simulink model "mrefrobotarm_previous_y_previous_u_previous_ref_cex_3"  (R2018b)
settings: Solver=FixedStepAuto  StartTime=0.0  StopTime=20  RelTol=1e-3  AbsTol=1e-6
undefined symbols (not defined in the file or in its folder): cc, options
libraries: neural x396, simulink x2
(part 7 of 15)

== system mrefrobotarm_previous_y_previous_u_previous_ref_cex_3/cex_m2_adapt/Layer 3/Delays 1 ==
  "p{3}" : Inport  PortDimensions=30
      mask Display: e = 0.06;c1 = [120 230 180]/255;c2 = ([120 230 180]+0)/(256+128);c3 = ([120 230 180]+128)/(256+128);patch([0 1 1 0],[0 0 1 1],c1);patch([0 1 1 1-e 1-e 0+e],[0 0 1 1-e 0+e 0+e],c2);patch([0 0 1 1-e 0+e 0+e],[0 1 1 1-e 1-e 0+e],c3);plot([0 1 1 0 0],[0 0 1 1 0]);
  mux : Mux  Inputs=1
      mask Display: e = 0.06;c1 = [120 150 230]/255;c2 = ([120 150 230]+0)/383;c3 = ([120 150 230]+128)/383;patch([0 1 1 0],[0 0 1 1],c1);patch([0 1 1 1-e 1-e 0+e],[0 0 1 1-e 0+e 0+e],c2);patch([0 0 1 1-e 0+e 0+e],[0 1 1 1-e 1-e 0+e],c3);plot([0 1 1 0 0],[0 0 1 1 0]);disp('Mux')
  "pd{3,2}" : Outport
      mask Display: e = 0.06;c1 = [120 230 180]/255;c2 = ([120 230 180]+0)/(256+128);c3 = ([120 230 180]+128)/(256+128);patch([0 1 1 0],[0 0 1 1],c1);patch([0 1 1 1-e 1-e 0+e],[0 0 1 1-e 0+e 0+e],c2);patch([0 0 1 1-e 0+e 0+e],[0 1 1 1-e 1-e 0+e],c3);plot([0 1 1 0 0],[0 0 1 1 0]);
  wires:
  "p{3}"/1 -> mux/1
  mux/1 -> "pd{3,2}"/1

== system mrefrobotarm_previous_y_previous_u_previous_ref_cex_3/cex_m2_adapt/Layer 3/LW{3,2} ==
  "ad{3,2}" : Inport  PortDimensions=30
      mask Display: e = 0.06;c1 = [120 230 180]/255;c2 = ([120 230 180]+0)/(256+128);c3 = ([120 230 180]+128)/(256+128);patch([0 1 1 0],[0 0 1 1],c1);patch([0 1 1 1-e 1-e 0+e],[0 0 1 1-e 0+e 0+e],c2);patch([0 0 1 1-e 0+e 0+e],[0 1 1 1-e 1-e 0+e],c3);plot([0 1 1 0 0],[0 0 1 1 0]);
  "IW{3,2}(1,:)'" : Constant  Value=[-0.05505125570900899767412539631550316698849201202392578125;-0.32891261733908494502287567229359410703182220458984375;0.415382135802389473866469415952451527118682861328125;-0.2282730838579582754999108828997123055160045623779296875;0.166865414887934881971176537263090722262859344482421875;-0.28767207852958420755129509416292421519756317138671875;-0.321285823362595035490585360093973577022552490234375;0.1207160846177025848025010645869770087301731109619140625;-0.01460446132137031838293950158913503400981426239013671875;0.5016492750276049239488429520861245691776275634765625;0.357718762934432665812067853039479814469814300537109375;-0.006297882074193773827008868693155818618834018707275390625;-0.0450799800946801443313205481899785809218883514404296875;0.0099702407715112732755624591618470731191337108612060546875;0.285267027442495102462771683349274098873138427734375;0.2491387260000068604171019615023396909236907958984375;-0.1838273412419492991443092932968284003436565399169921875;0.459873080865493555347001120026106946170330047607421875;0.036965404262347324737536524708048091270029544830322265625;0.038819216468767563099628858935830066911876201629638671875;0.320204321153936266597384019405581057071685791015625;-0.0222015075110175881534235742265082080848515033721923828125;0.1764216096534496347469911370353656820952892303466796875;-0.36905645815071663751183450585813261568546295166015625;-0.029660070230276454339435332485663820989429950714111328125;-0.036545858611714283903371125461490009911358356475830078125;0.2780670093635304596091373241506516933441162109375;0.5598975676846238425099500091164372861385345458984375;-0.217836892233410794883496919283061288297176361083984375;0.406407184848614377870035241357982158660888671875]
      mask Display: e = 0.06;c1 = [120 150 230]/255;c2 = ([120 150 230]+0)/383;c3 = ([120 150 230]+128)/383;patch([0 1 1 0],[0 0 1 1],c1);patch([0 1 1 1-e 1-e 0+e],[0 0 1 1-e 0+e 0+e],c2);patch([0 0 1 1-e 0+e 0+e],[0 1 1 1-e 1-e 0+e],c3);plot([0 1 1 0 0],[0 0 1 1 0]);disp('weights');
  Mux : Mux  Inputs=1
      mask Display: e = 0.06;c1 = [120 150 230]/255;c2 = ([120 150 230]+0)/383;c3 = ([120 150 230]+128)/383;patch([0 1 1 0],[0 0 1 1],c1);patch([0 1 1 1-e 1-e 0+e],[0 0 1 1-e 0+e 0+e],c2);patch([0 0 1 1-e 0+e 0+e],[0 1 1 1-e 1-e 0+e],c3);plot([0 1 1 0 0],[0 0 1 1 0]);disp('Mux');
  dotprod1 : neural/Weight Functions/dotprod
  "lz{3,2}" : Outport
      mask Display: e = 0.06;c1 = [120 230 180]/255;c2 = ([120 230 180]+0)/(256+128);c3 = ([120 230 180]+128)/(256+128);patch([0 1 1 0],[0 0 1 1],c1);patch([0 1 1 1-e 1-e 0+e],[0 0 1 1-e 0+e 0+e],c2);patch([0 0 1 1-e 0+e 0+e],[0 1 1 1-e 1-e 0+e],c3);plot([0 1 1 0 0],[0 0 1 1 0]);
  wires:
  "IW{3,2}(1,:)'"/1 -> dotprod1/1
  "ad{3,2}"/1 -> dotprod1/2
  dotprod1/1 -> Mux/1
  Mux/1 -> "lz{3,2}"/1

== system mrefrobotarm_previous_y_previous_u_previous_ref_cex_3/cex_m3_adapt/Layer 1/Delays 1 ==
  "p{1}" : Inport  PortDimensions=10
      mask Display: e = 0.06;c1 = [120 230 180]/255;c2 = ([120 230 180]+0)/(256+128);c3 = ([120 230 180]+128)/(256+128);patch([0 1 1 0],[0 0 1 1],c1);patch([0 1 1 1-e 1-e 0+e],[0 0 1 1-e 0+e 0+e],c2);patch([0 0 1 1-e 0+e 0+e],[0 1 1 1-e 1-e 0+e],c3);plot([0 1 1 0 0],[0 0 1 1 0]);
  mux : Mux  Inputs=1
      mask Display: e = 0.06;c1 = [120 150 230]/255;c2 = ([120 150 230]+0)/383;c3 = ([120 150 230]+128)/383;patch([0 1 1 0],[0 0 1 1],c1);patch([0 1 1 1-e 1-e 0+e],[0 0 1 1-e 0+e 0+e],c2);patch([0 0 1 1-e 0+e 0+e],[0 1 1 1-e 1-e 0+e],c3);plot([0 1 1 0 0],[0 0 1 1 0]);disp('Mux')
  "pd{1,1}" : Outport
      mask Display: e = 0.06;c1 = [120 230 180]/255;c2 = ([120 230 180]+0)/(256+128);c3 = ([120 230 180]+128)/(256+128);patch([0 1 1 0],[0 0 1 1],c1);patch([0 1 1 1-e 1-e 0+e],[0 0 1 1-e 0+e 0+e],c2);patch([0 0 1 1-e 0+e 0+e],[0 1 1 1-e 1-e 0+e],c3);plot([0 1 1 0 0],[0 0 1 1 0]);
  wires:
  "p{1}"/1 -> mux/1
  mux/1 -> "pd{1,1}"/1

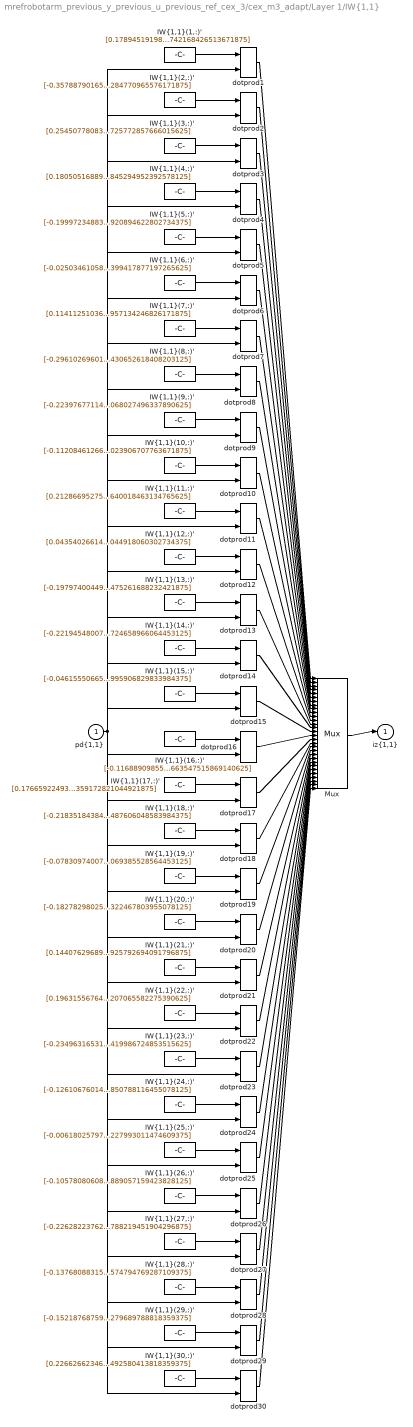
== system mrefrobotarm_previous_y_previous_u_previous_ref_cex_3/cex_m3_adapt/Layer 1/IW{1,1} ==
  "pd{1,1}" : Inport  PortDimensions=10
      mask Display: e = 0.06;c1 = [120 230 180]/255;c2 = ([120 230 180]+0)/(256+128);c3 = ([120 230 180]+128)/(256+128);patch([0 1 1 0],[0 0 1 1],c1);patch([0 1 1 1-e 1-e 0+e],[0 0 1 1-e 0+e 0+e],c2);patch([0 0 1 1-e 0+e 0+e],[0 1 1 1-e 1-e 0+e],c3);plot([0 1 1 0 0],[0 0 1 1 0]);
  "IW{1,1}(1,:)'" : Constant  Value=[0.178945191981768558786569656149367801845073699951171875;0.0268084580163748913139709628694618004374206066131591796875;-0.01942320989874750380987933340293238870799541473388671875;-0.08160193884960249832705159178658504970371723175048828125;-0.09141040548628250050899879397547920234501361846923828125;-0.03003006458415546919837879613623954355716705322265625;-0.2824185437874746629205446879495866596698760986328125;0.13111273715930271688279162844992242753505706787109375;-0.18958976093589396949568026684573851525783538818359375;0.2425037970369951778604189485122333280742168426513671875]
      mask Display: e = 0.06;c1 = [120 150 230]/255;c2 = ([120 150 230]+0)/383;c3 = ([120 150 230]+128)/383;patch([0 1 1 0],[0 0 1 1],c1);patch([0 1 1 1-e 1-e 0+e],[0 0 1 1-e 0+e 0+e],c2);patch([0 0 1 1-e 0+e 0+e],[0 1 1 1-e 1-e 0+e],c3);plot([0 1 1 0 0],[0 0 1 1 0]);disp('Weights');
  "IW{1,1}(10,:)'" : Constant  Value=[-0.11208461266883167073427074456049012951552867889404296875;0.357118226286030460148168685918790288269519805908203125;-0.2471912861743887079857273647576221264898777008056640625;0.02694087701823717762028564948195707984268665313720703125;0.333344688343605366487309993317467160522937774658203125;-0.3923720531710868097974298507324419915676116943359375;0.10448361375716642973632275470663444139063358306884765625;-0.06700094235100791106862772039676201529800891876220703125;-0.0864068226303956465894628991009085439145565032958984375;-0.39109116979221425491886066083679907023906707763671875]
      mask Display: e = 0.06;c1 = [120 150 230]/255;c2 = ([120 150 230]+0)/383;c3 = ([120 150 230]+128)/383;patch([0 1 1 0],[0 0 1 1],c1);patch([0 1 1 1-e 1-e 0+e],[0 0 1 1-e 0+e 0+e],c2);patch([0 0 1 1-e 0+e 0+e],[0 1 1 1-e 1-e 0+e],c3);plot([0 1 1 0 0],[0 0 1 1 0]);disp('Weights');
  "IW{1,1}(11,:)'" : Constant  Value=[0.2128669527513860348921781451281276531517505645751953125;-0.2022164608257241702471418420827831141650676727294921875;0.024891361043484862280994462935268529690802097320556640625;-0.1523659720349933854866009141915128566324710845947265625;0.01343407208234892631637524829102403600700199604034423828125;0.333788117058362920896996683950419537723064422607421875;-0.12203835126155791745983236751271761022508144378662109375;0.154459927321787870990732471909723244607448577880859375;-0.0299672295637235762411076933631193242035806179046630859375;0.1513977074327107763540567475502029992640018463134765625]
      mask Display: e = 0.06;c1 = [120 150 230]/255;c2 = ([120 150 230]+0)/383;c3 = ([120 150 230]+128)/383;patch([0 1 1 0],[0 0 1 1],c1);patch([0 1 1 1-e 1-e 0+e],[0 0 1 1-e 0+e 0+e],c2);patch([0 0 1 1-e 0+e 0+e],[0 1 1 1-e 1-e 0+e],c3);plot([0 1 1 0 0],[0 0 1 1 0]);disp('Weights');
  "IW{1,1}(12,:)'" : Constant  Value=[0.043540266140519097437522333393644657917320728302001953125;-0.41452389872784956015294710596208460628986358642578125;0.2152802602883765181740471916782553307712078094482421875;0.1665741110113748979504322278444305993616580963134765625;-0.02357125033996217144949270050346967764198780059814453125;0.0857396390633823612947850278942496515810489654541015625;-0.195803542101584737711306161145330406725406646728515625;-0.1624956920043294505973108243779279291629791259765625;0.251216496349794427001000940435915254056453704833984375;-0.10692808582410960605013627855441882275044918060302734375]
      mask Display: e = 0.06;c1 = [120 150 230]/255;c2 = ([120 150 230]+0)/383;c3 = ([120 150 230]+128)/383;patch([0 1 1 0],[0 0 1 1],c1);patch([0 1 1 1-e 1-e 0+e],[0 0 1 1-e 0+e 0+e],c2);patch([0 0 1 1-e 0+e 0+e],[0 1 1 1-e 1-e 0+e],c3);plot([0 1 1 0 0],[0 0 1 1 0]);disp('Weights');
  "IW{1,1}(13,:)'" : Constant  Value=[-0.197974004496612343562134128660545684397220611572265625;0.1845410275017112244899664119657245464622974395751953125;-0.06383715487094511475962832491859444417059421539306640625;0.212121113393368199151467479168786667287349700927734375;-0.13808972121742824068491017897031269967555999755859375;0.038970279682366611162525060763073270209133625030517578125;0.105618059669576991321804371182224713265895843505859375;-0.1502222390986265032619684234305168502032756805419921875;-0.24632715103327262884391757324920035898685455322265625;0.2171770229910456873057000848348252475261688232421875]
      mask Display: e = 0.06;c1 = [120 150 230]/255;c2 = ([120 150 230]+0)/383;c3 = ([120 150 230]+128)/383;patch([0 1 1 0],[0 0 1 1],c1);patch([0 1 1 1-e 1-e 0+e],[0 0 1 1-e 0+e 0+e],c2);patch([0 0 1 1-e 0+e 0+e],[0 1 1 1-e 1-e 0+e],c3);plot([0 1 1 0 0],[0 0 1 1 0]);disp('Weights');
  "IW{1,1}(14,:)'" : Constant  Value=[-0.2219454800708457742342005758473533205687999725341796875;-0.0314615502081657949506876548184663988649845123291015625;0.251007339093214987268964932809467427432537078857421875;-0.0716759461367137695742002279075677506625652313232421875;-0.0172769229951700541147996403879005811177194118499755859375;0.1873159588626435445579687666395329870283603668212890625;0.190073886084198784285348438061191700398921966552734375;0.256287607810354589599199925942230038344860076904296875;-0.12311553026235876051597273317383951507508754730224609375;0.08368773604129982335297910367444274015724658966064453125]
      mask Display: e = 0.06;c1 = [120 150 230]/255;c2 = ([120 150 230]+0)/383;c3 = ([120 150 230]+128)/383;patch([0 1 1 0],[0 0 1 1],c1);patch([0 1 1 1-e 1-e 0+e],[0 0 1 1-e 0+e 0+e],c2);patch([0 0 1 1-e 0+e 0+e],[0 1 1 1-e 1-e 0+e],c3);plot([0 1 1 0 0],[0 0 1 1 0]);disp('Weights');
  "IW{1,1}(15,:)'" : Constant  Value=[-0.046155506650369430843294793476161430589854717254638671875;-0.1501346179631337929283318999296170659363269805908203125;0.0092307094765049883811069975081409211270511150360107421875;-0.263036000331381802919139545338111929595470428466796875;-0.2327975024204980425412969680110109038650989532470703125;-0.2026112126291482462558946053832187317311763763427734375;0.051737301403803448440754664261476136744022369384765625;-0.209756826452610234401419120331411249935626983642578125;0.1810701775696283988281720667146146297454833984375;-0.037977678064883800546081005222731619141995906829833984375]
      mask Display: e = 0.06;c1 = [120 150 230]/255;c2 = ([120 150 230]+0)/383;c3 = ([120 150 230]+128)/383;patch([0 1 1 0],[0 0 1 1],c1);patch([0 1 1 1-e 1-e 0+e],[0 0 1 1-e 0+e 0+e],c2);patch([0 0 1 1-e 0+e 0+e],[0 1 1 1-e 1-e 0+e],c3);plot([0 1 1 0 0],[0 0 1 1 0]);disp('Weights');
  "IW{1,1}(16,:)'" : Constant  Value=[-0.11688909855486113997802277708615292795002460479736328125;0.1948288754210096562768939065790618769824504852294921875;0.245145418046943730505660141716361977159976959228515625;0.06314581600642978076454170377473928965628147125244140625;-0.1710702295590592336704816034398390911519527435302734375;0.2286371699946944946457705327702569775283336639404296875;0.1679562205641119965182639361955807544291019439697265625;-0.136021170064964225243642204077332280576229095458984375;0.1710849460743354699676643804195919074118137359619140625;-0.035177187616954430637861150898970663547515869140625]
      mask Display: e = 0.06;c1 = [120 150 230]/255;c2 = ([120 150 230]+0)/383;c3 = ([120 150 230]+128)/383;patch([0 1 1 0],[0 0 1 1],c1);patch([0 1 1 1-e 1-e 0+e],[0 0 1 1-e 0+e 0+e],c2);patch([0 0 1 1-e 0+e 0+e],[0 1 1 1-e 1-e 0+e],c3);plot([0 1 1 0 0],[0 0 1 1 0]);disp('Weights');
  "IW{1,1}(17,:)'" : Constant  Value=[0.1766592249333858999360558073021820746362209320068359375;-0.079243523014492278644382849961402826011180877685546875;-0.0793114419622731048331587544453213922679424285888671875;-0.1959259597757977700016596145360381342470645904541015625;0.11564958667334186703801179874062654562294483184814453125;0.0078762918190796345208060103004754637368023395538330078125;0.042690054177657914269428118814175832085311412811279296875;-0.209400363475176154448575971400714479386806488037109375;-0.1737241496218795144823587861537816934287548065185546875;-0.30776352047767552289059267422999255359172821044921875]
      mask Display: e = 0.06;c1 = [120 150 230]/255;c2 = ([120 150 230]+0)/383;c3 = ([120 150 230]+128)/383;patch([0 1 1 0],[0 0 1 1],c1);patch([0 1 1 1-e 1-e 0+e],[0 0 1 1-e 0+e 0+e],c2);patch([0 0 1 1-e 0+e 0+e],[0 1 1 1-e 1-e 0+e],c3);plot([0 1 1 0 0],[0 0 1 1 0]);disp('Weights');
  "IW{1,1}(18,:)'" : Constant  Value=[-0.21835184384607442265036070239148102700710296630859375;0.06422592695237487603332482422047178260982036590576171875;-0.061954335238517045658657167450655833818018436431884765625;0.09804573861090604136592219219892285764217376708984375;-0.1940740141485696457213094845428713597357273101806640625;0.1005519891302661117382655220353626646101474761962890625;0.05512324942271966399243154910436714999377727508544921875;-0.2225722743997785302294545317636220715939998626708984375;0.3076953257419956511142800081870518624782562255859375;0.03510283654959012178409238913445733487606048583984375]
      mask Display: e = 0.06;c1 = [120 150 230]/255;c2 = ([120 150 230]+0)/383;c3 = ([120 150 230]+128)/383;patch([0 1 1 0],[0 0 1 1],c1);patch([0 1 1 1-e 1-e 0+e],[0 0 1 1-e 0+e 0+e],c2);patch([0 0 1 1-e 0+e 0+e],[0 1 1 1-e 1-e 0+e],c3);plot([0 1 1 0 0],[0 0 1 1 0]);disp('Weights');
  "IW{1,1}(19,:)'" : Constant  Value=[-0.07830974007872003317398679200778133235871791839599609375;-0.11016442094929913830814172115424298681318759918212890625;0.0703650635811621516513270080395159311592578887939453125;-0.07372103454447127834914255117837456054985523223876953125;0.24983208769968501261615756448009051382541656494140625;-0.144793585299214433437242632862762548029422760009765625;0.321295391447031286613622569348081015050411224365234375;0.01420628885393082109500628718024017871357500553131103515625;-0.20975856453201091600391237079747952520847320556640625;-0.13789742091780443633552977189538069069385528564453125]
      mask Display: e = 0.06;c1 = [120 150 230]/255;c2 = ([120 150 230]+0)/383;c3 = ([120 150 230]+128)/383;patch([0 1 1 0],[0 0 1 1],c1);patch([0 1 1 1-e 1-e 0+e],[0 0 1 1-e 0+e 0+e],c2);patch([0 0 1 1-e 0+e 0+e],[0 1 1 1-e 1-e 0+e],c3);plot([0 1 1 0 0],[0 0 1 1 0]);disp('Weights');
  "IW{1,1}(2,:)'" : Constant  Value=[-0.357887901653798190526600819794111885130405426025390625;-0.1701515671788660366559042813605628907680511474609375;0.1283989037480392225720748911044211126863956451416015625;0.02788164361507915189886119833317934535443782806396484375;0.2413361422270965395142638953984715044498443603515625;-0.088300044465701998941398187525919638574123382568359375;-0.059645869356086879398137767793741659261286258697509765625;-0.1817714760329936229954483906112727709114551544189453125;-0.2027513482131242106287771775896544568240642547607421875;0.0361216702772399755883014904611627571284770965576171875]
      mask Display: e = 0.06;c1 = [120 150 230]/255;c2 = ([120 150 230]+0)/383;c3 = ([120 150 230]+128)/383;patch([0 1 1 0],[0 0 1 1],c1);patch([0 1 1 1-e 1-e 0+e],[0 0 1 1-e 0+e 0+e],c2);patch([0 0 1 1-e 0+e 0+e],[0 1 1 1-e 1-e 0+e],c3);plot([0 1 1 0 0],[0 0 1 1 0]);disp('Weights');
  "IW{1,1}(20,:)'" : Constant  Value=[-0.1827829802579581663923846690522623248398303985595703125;0.429762651162807263194309825848904438316822052001953125;0.047505038489587501915334399882340221665799617767333984375;-0.051722345762055088602693331267801113426685333251953125;0.09193146508099292457671936062979511916637420654296875;-0.378843620454603124958481430439860559999942779541015625;-0.0326607967189324333023847657386795617640018463134765625;-0.035941474259534145208050404107780195772647857666015625;-0.0821945981870604303054506090120412409305572509765625;-0.1229102528711117081616777113595162518322467803955078125]
      mask Display: e = 0.06;c1 = [120 150 230]/255;c2 = ([120 150 230]+0)/383;c3 = ([120 150 230]+128)/383;patch([0 1 1 0],[0 0 1 1],c1);patch([0 1 1 1-e 1-e 0+e],[0 0 1 1-e 0+e 0+e],c2);patch([0 0 1 1-e 0+e 0+e],[0 1 1 1-e 1-e 0+e],c3);plot([0 1 1 0 0],[0 0 1 1 0]);disp('Weights');
  "IW{1,1}(21,:)'" : Constant  Value=[0.1440762968925218545646060874787508510053157806396484375;0.0567506407928204670287897215530392713844776153564453125;0.18700116751710360585292391988332383334636688232421875;-0.1647839415001810803307336072975886054337024688720703125;-0.237372168308809750048027353841462172567844390869140625;0.253696421920278913919588603675947524607181549072265625;-0.2346470875872900541114773886874900199472904205322265625;0.0215979693524790301861759900248216581530869007110595703125;0.23838840468809874284517036358010955154895782470703125;-0.0025999808583438833824164060359862560289911925792694091796875]
      mask Display: e = 0.06;c1 = [120 150 230]/255;c2 = ([120 150 230]+0)/383;c3 = ([120 150 230]+128)/383;patch([0 1 1 0],[0 0 1 1],c1);patch([0 1 1 1-e 1-e 0+e],[0 0 1 1-e 0+e 0+e],c2);patch([0 0 1 1-e 0+e 0+e],[0 1 1 1-e 1-e 0+e],c3);plot([0 1 1 0 0],[0 0 1 1 0]);disp('Weights');
  "IW{1,1}(22,:)'" : Constant  Value=[0.1963155676454732267988134708502911962568759918212890625;-0.052000800150651706188487111148788244463503360748291015625;-0.271534817188853139224846700017224065959453582763671875;-0.0895242263296035234443337458287714980542659759521484375;-0.03695111731571724955625057873476180247962474822998046875;0.004478426352357927318903474400713093928061425685882568359375;0.259203736873355072845015456550754606723785400390625;-0.08894384724343833148463289717255975119769573211669921875;0.0322689444357559251930211985381902195513248443603515625;0.306951155849270629349945238573127426207065582275390625]
      mask Display: e = 0.06;c1 = [120 150 230]/255;c2 = ([120 150 230]+0)/383;c3 = ([120 150 230]+128)/383;patch([0 1 1 0],[0 0 1 1],c1);patch([0 1 1 1-e 1-e 0+e],[0 0 1 1-e 0+e 0+e],c2);patch([0 0 1 1-e 0+e 0+e],[0 1 1 1-e 1-e 0+e],c3);plot([0 1 1 0 0],[0 0 1 1 0]);disp('Weights');
  "IW{1,1}(23,:)'" : Constant  Value=[-0.2349631653173517020771754459929070435464382171630859375;-0.17641432489103936465113520171144045889377593994140625;0.234912163501337811766234153765253722667694091796875;0.09797598509365797181391855019683134742081165313720703125;0.27541255175971579571836400646134279668331146240234375;-0.006673026099757165506554112965886815800331532955169677734375;-0.08630883651204894480013507518378901295363903045654296875;-0.0492544357827646994696380033929017372429370880126953125;0.3119811671615313475314223978784866631031036376953125;-0.1301709266317944424518060486661852337419986724853515625]
      mask Display: e = 0.06;c1 = [120 150 230]/255;c2 = ([120 150 230]+0)/383;c3 = ([120 150 230]+128)/383;patch([0 1 1 0],[0 0 1 1],c1);patch([0 1 1 1-e 1-e 0+e],[0 0 1 1-e 0+e 0+e],c2);patch([0 0 1 1-e 0+e 0+e],[0 1 1 1-e 1-e 0+e],c3);plot([0 1 1 0 0],[0 0 1 1 0]);disp('Weights');
  "IW{1,1}(24,:)'" : Constant  Value=[-0.126106760142745744079917358249076642096042633056640625;0.08453625577713620720121667773128137923777103424072265625;-0.1709608100596076152299929162836633622646331787109375;0.291185745152728825413390723042539320886135101318359375;0.11522508174914349032835758634973899461328983306884765625;0.270251365920760211469797695826855488121509552001953125;0.11501887877284679151390633933260687626898288726806640625;0.068932792124765829289145813163486309349536895751953125;0.0923120543919047076286688024993054568767547607421875;0.12574612443187327404103825756465084850788116455078125]
      mask Display: e = 0.06;c1 = [120 150 230]/255;c2 = ([120 150 230]+0)/383;c3 = ([120 150 230]+128)/383;patch([0 1 1 0],[0 0 1 1],c1);patch([0 1 1 1-e 1-e 0+e],[0 0 1 1-e 0+e 0+e],c2);patch([0 0 1 1-e 0+e 0+e],[0 1 1 1-e 1-e 0+e],c3);plot([0 1 1 0 0],[0 0 1 1 0]);disp('Weights');
  "IW{1,1}(25,:)'" : Constant  Value=[-0.00618025797029859470799184606448761769570410251617431640625;0.1585465053945979418958955875496030785143375396728515625;0.1885969000154264219037969496639561839401721954345703125;-0.0168828019608085848346501478545178542844951152801513671875;-0.1887944529566672191567278105139848776161670684814453125;0.127242314587684257620736616445356048643589019775390625;-0.0185715628598672015392434531122489715926349163055419921875;0.271969474158978596900482216369709931313991546630859375;0.11406243308473180964046633789621409960091114044189453125;-0.2380937855451320250832480951430625282227993011474609375]
      mask Display: e = 0.06;c1 = [120 150 230]/255;c2 = ([120 150 230]+0)/383;c3 = ([120 150 230]+128)/383;patch([0 1 1 0],[0 0 1 1],c1);patch([0 1 1 1-e 1-e 0+e],[0 0 1 1-e 0+e 0+e],c2);patch([0 0 1 1-e 0+e 0+e],[0 1 1 1-e 1-e 0+e],c3);plot([0 1 1 0 0],[0 0 1 1 0]);disp('Weights');
  "IW{1,1}(26,:)'" : Constant  Value=[-0.1057808060816034234630222954365308396518230438232421875;0.1781977064655418108163331680771079845726490020751953125;-0.25777667563861805799518833737238310277462005615234375;-0.12119534915408673725334409709830651991069316864013671875;0.107985561966510490439219438485451973974704742431640625;0.032407409608050032068238266447224305011332035064697265625;0.233920314605909063221389487807755358517169952392578125;0.04861961739534488569081105424629640765488147735595703125;-0.07777090296223808374431740730869933031499385833740234375;-0.06606828886995681771043820162958581931889057159423828125]
      mask Display: e = 0.06;c1 = [120 150 230]/255;c2 = ([120 150 230]+0)/383;c3 = ([120 150 230]+128)/383;patch([0 1 1 0],[0 0 1 1],c1);patch([0 1 1 1-e 1-e 0+e],[0 0 1 1-e 0+e 0+e],c2);patch([0 0 1 1-e 0+e 0+e],[0 1 1 1-e 1-e 0+e],c3);plot([0 1 1 0 0],[0 0 1 1 0]);disp('Weights');
  "IW{1,1}(27,:)'" : Constant  Value=[-0.2262822376263129708906518544608843512833118438720703125;0.228376340453633808191824527966673485934734344482421875;-0.04633621010046702626272718816835549660027027130126953125;-0.21557195704307108297115291861700825393199920654296875;-0.024477301255473281338392865791320218704640865325927734375;-0.061316063341058886504431058028785628266632556915283203125;0.19263265023581077617365053811226971447467803955078125;0.21379549598064950810538675796124152839183807373046875;0.2402192329457557284921875861982698552310466766357421875;0.004684371003340066612341541230080110835842788219451904296875]
      mask Display: e = 0.06;c1 = [120 150 230]/255;c2 = ([120 150 230]+0)/383;c3 = ([120 150 230]+128)/383;patch([0 1 1 0],[0 0 1 1],c1);patch([0 1 1 1-e 1-e 0+e],[0 0 1 1-e 0+e 0+e],c2);patch([0 0 1 1-e 0+e 0+e],[0 1 1 1-e 1-e 0+e],c3);plot([0 1 1 0 0],[0 0 1 1 0]);disp('Weights');
  "IW{1,1}(28,:)'" : Constant  Value=[-0.137680883158168343438632064135163091123104095458984375;0.1357222867627534690360135982700739987194538116455078125;0.10901823944261945786848855277639813721179962158203125;-0.0209386438839303558323567955312682897783815860748291015625;0.1596112896660535629411725722093251533806324005126953125;-0.224640567202143426328575515071861445903778076171875;-0.126750799819497272924451181097538210451602935791015625;0.1520166458419669186508116354161757044494152069091796875;0.21814044502030494054878317911061458289623260498046875;-0.04722597981823682677937625840058899484574794769287109375]
      mask Display: e = 0.06;c1 = [120 150 230]/255;c2 = ([120 150 230]+0)/383;c3 = ([120 150 230]+128)/383;patch([0 1 1 0],[0 0 1 1],c1);patch([0 1 1 1-e 1-e 0+e],[0 0 1 1-e 0+e 0+e],c2);patch([0 0 1 1-e 0+e 0+e],[0 1 1 1-e 1-e 0+e],c3);plot([0 1 1 0 0],[0 0 1 1 0]);disp('Weights');
  "IW{1,1}(29,:)'" : Constant  Value=[-0.152187687592834297589661218808032572269439697265625;-0.045824332750618645970774878151132725179195404052734375;0.0755527612060038489261160066234879195690155029296875;-0.185261645573886746252156854097847826778888702392578125;0.1512516263026323082296897837295546196401119232177734375;-0.1412085300290002454204341120203025639057159423828125;-0.0868175921655288396205918388659483753144741058349609375;-0.2248728415417697579226086190828937105834484100341796875;-0.1651996539641483463523030650321743451058864593505859375;0.15755372160029990080687412046245299279689788818359375]
      mask Display: e = 0.06;c1 = [120 150 230]/255;c2 = ([120 150 230]+0)/383;c3 = ([120 150 230]+128)/383;patch([0 1 1 0],[0 0 1 1],c1);patch([0 1 1 1-e 1-e 0+e],[0 0 1 1-e 0+e 0+e],c2);patch([0 0 1 1-e 0+e 0+e],[0 1 1 1-e 1-e 0+e],c3);plot([0 1 1 0 0],[0 0 1 1 0]);disp('Weights');
  "IW{1,1}(3,:)'" : Constant  Value=[0.2545077808367981475612396025098860263824462890625;0.040200788949858144716298369303331128321588039398193359375;0.16885529405137200686937148930155672132968902587890625;0.2275439655005222217010185659091803245246410369873046875;0.238416395262542712973896641415194608271121978759765625;0.1413290820820835846927110424076090566813945770263671875;0.10575858892024310453638946682985988445580005645751953125;0.13340769511394778845669861766509711742401123046875;0.12030518096117114035248363279606564901769161224365234375;0.1159861633997042729138371441877097822725772857666015625]
      mask Display: e = 0.06;c1 = [120 150 230]/255;c2 = ([120 150 230]+0)/383;c3 = ([120 150 230]+128)/383;patch([0 1 1 0],[0 0 1 1],c1);patch([0 1 1 1-e 1-e 0+e],[0 0 1 1-e 0+e 0+e],c2);patch([0 0 1 1-e 0+e 0+e],[0 1 1 1-e 1-e 0+e],c3);plot([0 1 1 0 0],[0 0 1 1 0]);disp('Weights');
  "IW{1,1}(30,:)'" : Constant  Value=[0.2266266234642653198960715599241666495800018310546875;0.1400900685113556087824093765448196791112422943115234375;-0.111869786415829397530075084432610310614109039306640625;0.2012524327790981004682180355302989482879638671875;-0.0186272552060192768397239859723413246683776378631591796875;-0.2006401151986405839711125054236617870628833770751953125;-0.09615820230093363729650945970206521451473236083984375;-0.1772150327736468355954713160826941020786762237548828125;0.031918350708111407898481814982005744241178035736083984375;0.26696557032662437958236978374770842492580413818359375]
      mask Display: e = 0.06;c1 = [120 150 230]/255;c2 = ([120 150 230]+0)/383;c3 = ([120 150 230]+128)/383;patch([0 1 1 0],[0 0 1 1],c1);patch([0 1 1 1-e 1-e 0+e],[0 0 1 1-e 0+e 0+e],c2);patch([0 0 1 1-e 0+e 0+e],[0 1 1 1-e 1-e 0+e],c3);plot([0 1 1 0 0],[0 0 1 1 0]);disp('Weights');
  "IW{1,1}(4,:)'" : Constant  Value=[0.1805051688978105695060349944469635374844074249267578125;-0.2288494814434568758176880010068998672068119049072265625;0.1818720593742958191452174787627882324159145355224609375;-0.037942953544057432535563378905862919054925441741943359375;-0.005389968593745760212787576648452159133739769458770751953125;0.1827951113605962019104111959677538834512233734130859375;-0.055292178726246830888779726365100941620767116546630859375;-0.14743556348991282423099846710101701319217681884765625;-0.2793310799565957847079289422254078090190887451171875;0.1322500450627073498299779430453781969845294952392578125]
      mask Display: e = 0.06;c1 = [120 150 230]/255;c2 = ([120 150 230]+0)/383;c3 = ([120 150 230]+128)/383;patch([0 1 1 0],[0 0 1 1],c1);patch([0 1 1 1-e 1-e 0+e],[0 0 1 1-e 0+e 0+e],c2);patch([0 0 1 1-e 0+e 0+e],[0 1 1 1-e 1-e 0+e],c3);plot([0 1 1 0 0],[0 0 1 1 0]);disp('Weights');
  "IW{1,1}(5,:)'" : Constant  Value=[-0.1999723488349300082322912430754513479769229888916015625;-0.16296175086491249128783920241403393447399139404296875;-0.10880631133516142916572988497136975638568401336669921875;0.051130749748494554174360615661498741246759891510009765625;-0.02372298130379191238858993528992868959903717041015625;0.0517192502525367914234522004335303790867328643798828125;-0.1720233138208674128488695487249060533940792083740234375;-0.204481799674667341637501749573857523500919342041015625;0.1663037664222504485866949153205496259033679962158203125;-0.139186530375922268287780525497510097920894622802734375]
      mask Display: e = 0.06;c1 = [120 150 230]/255;c2 = ([120 150 230]+0)/383;c3 = ([120 150 230]+128)/383;patch([0 1 1 0],[0 0 1 1],c1);patch([0 1 1 1-e 1-e 0+e],[0 0 1 1-e 0+e 0+e],c2);patch([0 0 1 1-e 0+e 0+e],[0 1 1 1-e 1-e 0+e],c3);plot([0 1 1 0 0],[0 0 1 1 0]);disp('Weights');
  "IW{1,1}(6,:)'" : Constant  Value=[-0.0250346105868364705859807628485214081592857837677001953125;-0.004457760763241335431883438644717898569069802761077880859375;0.0664046720124821521213931418969877995550632476806640625;-0.2130593218179563930192443876876495778560638427734375;0.1292973325083253133271909973700530827045440673828125;-0.1347766108497021608769728118204511702060699462890625;-0.235986082534269503430124359510955400764942169189453125;-0.0652885071425104157594176967904786579310894012451171875;-0.1443016385971503112717329031511326320469379425048828125;0.08876763803892606663481501527712680399417877197265625]
      mask Display: e = 0.06;c1 = [120 150 230]/255;c2 = ([120 150 230]+0)/383;c3 = ([120 150 230]+128)/383;patch([0 1 1 0],[0 0 1 1],c1);patch([0 1 1 1-e 1-e 0+e],[0 0 1 1-e 0+e 0+e],c2);patch([0 0 1 1-e 0+e 0+e],[0 1 1 1-e 1-e 0+e],c3);plot([0 1 1 0 0],[0 0 1 1 0]);disp('Weights');
  "IW{1,1}(7,:)'" : Constant  Value=[0.1141125103679923313837463183517684228718280792236328125;-0.071976397782599510488665828233934007585048675537109375;0.2194208546389509739693579604136175476014614105224609375;0.2087203652399640396719604495956446044147014617919921875;0.04279122020650989732803992637855117209255695343017578125;0.0121936683836014019000071328946432913653552532196044921875;0.10314941535816808670933397706903633661568164825439453125;0.215596517802053522228078463740530423820018768310546875;-0.11201446245962991266065245099525782279670238494873046875;0.267689612477664595768800381847540847957134246826171875]
      mask Display: e = 0.06;c1 = [120 150 230]/255;c2 = ([120 150 230]+0)/383;c3 = ([120 150 230]+128)/383;patch([0 1 1 0],[0 0 1 1],c1);patch([0 1 1 1-e 1-e 0+e],[0 0 1 1-e 0+e 0+e],c2);patch([0 0 1 1-e 0+e 0+e],[0 1 1 1-e 1-e 0+e],c3);plot([0 1 1 0 0],[0 0 1 1 0]);disp('Weights');
  "IW{1,1}(8,:)'" : Constant  Value=[-0.29610269601041749876202402447233907878398895263671875;-0.0746339250862548819753783391206525266170501708984375;-0.238554927372123748430254863706068135797977447509765625;-0.2056115987616206897126147623566794209182262420654296875;0.052565514438149885112494530403637327253818511962890625;-0.1454333409079378303108143200006452389061450958251953125;0.15678849503835790013539508436224423348903656005859375;0.172166717933729118694685666923760436475276947021484375;-0.0903178103674671384215599800882046110928058624267578125;-0.05251415724731541001535362056529265828430652618408203125]
      mask Display: e = 0.06;c1 = [120 150 230]/255;c2 = ([120 150 230]+0)/383;c3 = ([120 150 230]+128)/383;patch([0 1 1 0],[0 0 1 1],c1);patch([0 1 1 1-e 1-e 0+e],[0 0 1 1-e 0+e 0+e],c2);patch([0 0 1 1-e 0+e 0+e],[0 1 1 1-e 1-e 0+e],c3);plot([0 1 1 0 0],[0 0 1 1 0]);disp('Weights');
  "IW{1,1}(9,:)'" : Constant  Value=[-0.2239767711452672338534597429315908811986446380615234375;-0.1882927516835710413101168114735628478229045867919921875;-0.025793704558856107855735473322056350298225879669189453125;0.078152304715024045744797831503092311322689056396484375;0.035626975658994801399170881950340117327868938446044921875;-0.037320265281373166121881013168604113161563873291015625;-0.280711906735009508739864259041496552526950836181640625;0.326090669546220401908698249826557002961635589599609375;0.052075481844195310732192893965475377626717090606689453125;-0.0171626623121999034859985755474554025568068027496337890625]
      mask Display: e = 0.06;c1 = [120 150 230]/255;c2 = ([120 150 230]+0)/383;c3 = ([120 150 230]+128)/383;patch([0 1 1 0],[0 0 1 1],c1);patch([0 1 1 1-e 1-e 0+e],[0 0 1 1-e 0+e 0+e],c2);patch([0 0 1 1-e 0+e 0+e],[0 1 1 1-e 1-e 0+e],c3);plot([0 1 1 0 0],[0 0 1 1 0]);disp('Weights');
  Mux : Mux  Inputs=30
      mask Display: e = 0.06;c1 = [120 150 230]/255;c2 = ([120 150 230]+0)/383;c3 = ([120 150 230]+128)/383;patch([0 1 1 0],[0 0 1 1],c1);patch([0 1 1 1-e 1-e 0+e],[0 0 1 1-e 0+e 0+e],c2);patch([0 0 1 1-e 0+e 0+e],[0 1 1 1-e 1-e 0+e],c3);plot([0 1 1 0 0],[0 0 1 1 0]);disp('Mux');
  dotprod{1..30} (30 alike) : neural/Weight Functions/dotprod
  "iz{1,1}" : Outport
      mask Display: e = 0.06;c1 = [120 230 180]/255;c2 = ([120 230 180]+0)/(256+128);c3 = ([120 230 180]+128)/(256+128);patch([0 1 1 0],[0 0 1 1],c1);patch([0 1 1 1-e 1-e 0+e],[0 0 1 1-e 0+e 0+e],c2);patch([0 0 1 1-e 0+e 0+e],[0 1 1 1-e 1-e 0+e],c3);plot([0 1 1 0 0],[0 0 1 1 0]);
  wires:
  "IW{1,1}(1,:)'"/1 -> dotprod1/1
  "pd{1,1}"/1 -> dotprod1/2, dotprod2/2, dotprod3/2, dotprod4/2, dotprod5/2, dotprod6/2, dotprod7/2, dotprod8/2, dotprod9/2, dotprod10/2, dotprod11/2, dotprod12/2, dotprod13/2, dotprod14/2, dotprod15/2, dotprod16/2, dotprod17/2, dotprod18/2, dotprod19/2, dotprod20/2, dotprod21/2, dotprod22/2, dotprod23/2, dotprod24/2, dotprod25/2, dotprod26/2, dotprod27/2, dotprod28/2, dotprod29/2, dotprod30/2
  dotprod1/1 -> Mux/1
  "IW{1,1}(2,:)'"/1 -> dotprod2/1
  dotprod2/1 -> Mux/2
  "IW{1,1}(3,:)'"/1 -> dotprod3/1
  dotprod3/1 -> Mux/3
  "IW{1,1}(4,:)'"/1 -> dotprod4/1
  dotprod4/1 -> Mux/4
  "IW{1,1}(5,:)'"/1 -> dotprod5/1
  dotprod5/1 -> Mux/5
  "IW{1,1}(6,:)'"/1 -> dotprod6/1
  dotprod6/1 -> Mux/6
  "IW{1,1}(7,:)'"/1 -> dotprod7/1
  dotprod7/1 -> Mux/7
  "IW{1,1}(8,:)'"/1 -> dotprod8/1
  dotprod8/1 -> Mux/8
  "IW{1,1}(9,:)'"/1 -> dotprod9/1
  dotprod9/1 -> Mux/9
  "IW{1,1}(10,:)'"/1 -> dotprod10/1
  dotprod10/1 -> Mux/10
  "IW{1,1}(11,:)'"/1 -> dotprod11/1
  dotprod11/1 -> Mux/11
  "IW{1,1}(12,:)'"/1 -> dotprod12/1
  dotprod12/1 -> Mux/12
  "IW{1,1}(13,:)'"/1 -> dotprod13/1
  dotprod13/1 -> Mux/13
  "IW{1,1}(14,:)'"/1 -> dotprod14/1
  dotprod14/1 -> Mux/14
  "IW{1,1}(15,:)'"/1 -> dotprod15/1
  dotprod15/1 -> Mux/15
  "IW{1,1}(16,:)'"/1 -> dotprod16/1
  dotprod16/1 -> Mux/16
  "IW{1,1}(17,:)'"/1 -> dotprod17/1
  dotprod17/1 -> Mux/17
  "IW{1,1}(18,:)'"/1 -> dotprod18/1
  dotprod18/1 -> Mux/18
  "IW{1,1}(19,:)'"/1 -> dotprod19/1
  dotprod19/1 -> Mux/19
  "IW{1,1}(20,:)'"/1 -> dotprod20/1
  dotprod20/1 -> Mux/20
  "IW{1,1}(21,:)'"/1 -> dotprod21/1
  dotprod21/1 -> Mux/21
  "IW{1,1}(22,:)'"/1 -> dotprod22/1
  dotprod22/1 -> Mux/22
  "IW{1,1}(23,:)'"/1 -> dotprod23/1
  dotprod23/1 -> Mux/23
  "IW{1,1}(24,:)'"/1 -> dotprod24/1
  dotprod24/1 -> Mux/24
  "IW{1,1}(25,:)'"/1 -> dotprod25/1
  dotprod25/1 -> Mux/25
  "IW{1,1}(26,:)'"/1 -> dotprod26/1
  dotprod26/1 -> Mux/26
  "IW{1,1}(27,:)'"/1 -> dotprod27/1
  dotprod27/1 -> Mux/27
  "IW{1,1}(28,:)'"/1 -> dotprod28/1
  dotprod28/1 -> Mux/28
  "IW{1,1}(29,:)'"/1 -> dotprod29/1
  dotprod29/1 -> Mux/29
  "IW{1,1}(30,:)'"/1 -> dotprod30/1
  dotprod30/1 -> Mux/30
  Mux/1 -> "iz{1,1}"/1

== system mrefrobotarm_previous_y_previous_u_previous_ref_cex_3/cex_m3_adapt/Layer 2/Delays 1 ==
  "p{2}" : Inport  PortDimensions=30
      mask Display: e = 0.06;c1 = [120 230 180]/255;c2 = ([120 230 180]+0)/(256+128);c3 = ([120 230 180]+128)/(256+128);patch([0 1 1 0],[0 0 1 1],c1);patch([0 1 1 1-e 1-e 0+e],[0 0 1 1-e 0+e 0+e],c2);patch([0 0 1 1-e 0+e 0+e],[0 1 1 1-e 1-e 0+e],c3);plot([0 1 1 0 0],[0 0 1 1 0]);
  mux : Mux  Inputs=1
      mask Display: e = 0.06;c1 = [120 150 230]/255;c2 = ([120 150 230]+0)/383;c3 = ([120 150 230]+128)/383;patch([0 1 1 0],[0 0 1 1],c1);patch([0 1 1 1-e 1-e 0+e],[0 0 1 1-e 0+e 0+e],c2);patch([0 0 1 1-e 0+e 0+e],[0 1 1 1-e 1-e 0+e],c3);plot([0 1 1 0 0],[0 0 1 1 0]);disp('Mux')
  "pd{2,1}" : Outport
      mask Display: e = 0.06;c1 = [120 230 180]/255;c2 = ([120 230 180]+0)/(256+128);c3 = ([120 230 180]+128)/(256+128);patch([0 1 1 0],[0 0 1 1],c1);patch([0 1 1 1-e 1-e 0+e],[0 0 1 1-e 0+e 0+e],c2);patch([0 0 1 1-e 0+e 0+e],[0 1 1 1-e 1-e 0+e],c3);plot([0 1 1 0 0],[0 0 1 1 0]);
  wires:
  "p{2}"/1 -> mux/1
  mux/1 -> "pd{2,1}"/1
